simulink model "HVDC_VSC_1CPUcore_dcpl"  (Simulink 8.4)
settings: Solver=ode3  SolverMode=SingleTasking  StartTime=0.0  StopTime=70.0  FixedStep=Ts_Power  RelTol=1e-3  AbsTol=1e-2
PreLoadFcn:
  | Ts_Power=50e-6; Ts_Control=1*Ts_Power; init_cosim_IA; startup_transients_hvdc_vsc;
PostLoadFcn:
  | Ts_Power=50e-6; Ts_Control=1*Ts_Power; init_cosim_IA; startup_transients_hvdc_vsc;
InitFcn:
  | Ts_Power=50e-6; Ts_Control=1*Ts_Power; init_cosim_IA; startup_transients_hvdc_vsc;
values from neighbouring files (symbols this model uses):
  h = 5    [init_cosim_IA.m]
  intfDelay = 400.0    (= 400)    [init_cosim_IA.m]
  Ts_intf = 2*Ts_Power    [init_cosim_IA.m]
undefined symbols (not defined in the file or in its folder): CLARK, D1, Delta, dPref1_2, dPref1_2_rlimit, gcbh, level, lib_mesures, magnitude, ResistanceM, rte_drive_private_lib, rte_tsb3level_hiz_rect_cb, sps_rtmsupport, t_deblock_Pref1, t_deblock_Udref2, t_dPref1_2, t_init_AC, t_SwitchITMIdc, t_SwitchITMVdc, t_vsag_end, t_vsag_start, TSB3_hiZR
libraries: powerlib x162, powerlib_extras x71, spsVIMeasurementModel x63, rteventslib x26, op_dpl_lib x14, powerlib_meascontrol x14, rtlab x6, sps_avr x3, artemis x1
(part 2 of 11)

== system HVDC_VSC_1CPUcore_dcpl/SM_HVDC_VSC/37.5-km  cable ==
  Artemis DPL1 : Subsystem
  Artemis DPL2 : Subsystem
  BI : Subsystem  Tag=ARTEMIS model
      settings: AttributesFormatString=%<Tag>
  PM1 : PMIOPort  Port=1  Side=Left
  PM2 : PMIOPort  Port=2  Side=Right
  wires:
  Artemis DPL2/1(ho) -> Artemis DPL1/1(hi)
  Artemis DPL1/1(ho) -> Artemis DPL2/1(hi)
  connections:
  Artemis DPL2/LConn1 -- PM2/RConn1
  PM1/RConn1 -- Artemis DPL1/LConn1

== system HVDC_VSC_1CPUcore_dcpl/SM_HVDC_VSC/37.5-km  cable1 ==
  Artemis DPL1 : Subsystem
  Artemis DPL2 : Subsystem
  BI : Subsystem  Tag=ARTEMIS model
      settings: AttributesFormatString=%<Tag>
  PM1 : PMIOPort  Port=1  Side=Left
  PM2 : PMIOPort  Port=2  Side=Right
  wires:
  Artemis DPL1/1(ho) -> Artemis DPL2/1(hi)
  Artemis DPL2/1(ho) -> Artemis DPL1/1(hi)
  connections:
  PM1/RConn1 -- Artemis DPL1/LConn1
  Artemis DPL2/LConn1 -- PM2/RConn1

== system HVDC_VSC_1CPUcore_dcpl/SM_HVDC_VSC/37.5-km cable ==
  Artemis DPL1 : Subsystem
  Artemis DPL2 : Subsystem
  BI : Subsystem  Tag=ARTEMIS model
      settings: AttributesFormatString=%<Tag>
  PM1 : PMIOPort  Port=1  Side=Left
  PM2 : PMIOPort  Port=2  Side=Right
  wires:
  Artemis DPL1/1(ho) -> Artemis DPL2/1(hi)
  Artemis DPL2/1(ho) -> Artemis DPL1/1(hi)
  connections:
  PM1/RConn1 -- Artemis DPL1/LConn1
  Artemis DPL2/LConn1 -- PM2/RConn1

== system HVDC_VSC_1CPUcore_dcpl/SM_HVDC_VSC/37.5-km cable1 ==
  Artemis DPL1 : Subsystem
  Artemis DPL2 : Subsystem
  BI : Subsystem  Tag=ARTEMIS model
      settings: AttributesFormatString=%<Tag>
  PM1 : PMIOPort  Port=1  Side=Left
  PM2 : PMIOPort  Port=2  Side=Right
  wires:
  Artemis DPL2/1(ho) -> Artemis DPL1/1(hi)
  Artemis DPL1/1(ho) -> Artemis DPL2/1(hi)
  connections:
  Artemis DPL2/LConn1 -- PM2/RConn1
  PM1/RConn1 -- Artemis DPL1/LConn1

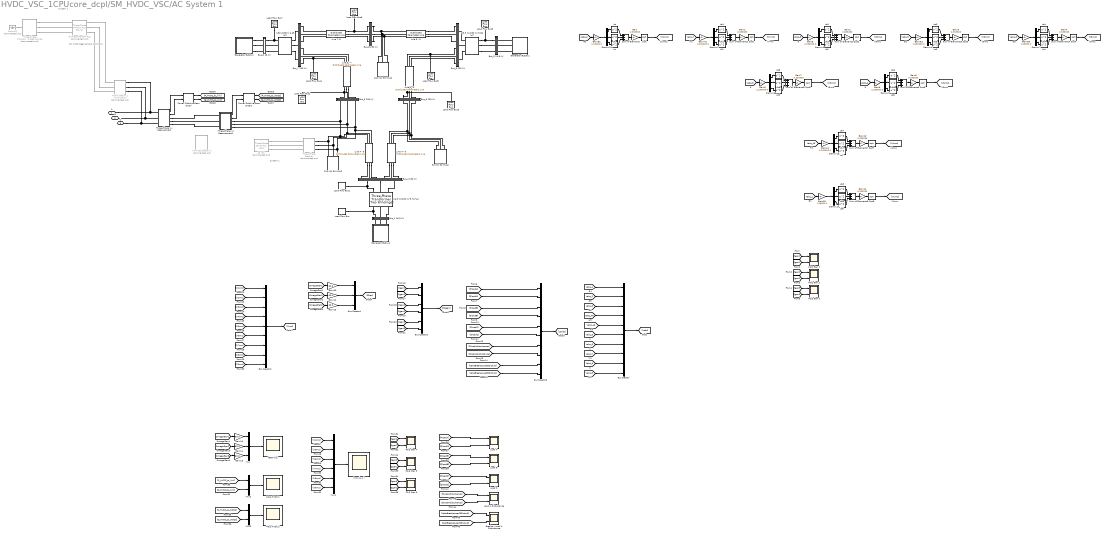
== system HVDC_VSC_1CPUcore_dcpl/SM_HVDC_VSC/AC System 1 ==
  note: phi = 80 (deg) at 1st & 3rd harm.
  note: System 1
  note: System 1
  " Line 4 - 6" : op_dpl_lib/Distributed Parameters Line  SimulationMode=ARTEMIS model  Phases=3  Frequency=60  Resistance=[0.08993 0.224825]  Inductance="[1.41e-3  3.22e-3]"  Capacitance=[7.922e-9 4.74e-9]  Length=100  Measurements=None
  " Line 6 - 9" : op_dpl_lib/Distributed Parameters Line  SimulationMode=ARTEMIS model  Phases=3  Frequency=60  Resistance=[0.20631 0.5157]  Inductance="[2.38e-3  6.09e-3]"  Capacitance=[17.95e-9 10.55e-9]  Length=100  Measurements=None
  100 MW 35 MVAR : powerlib/Elements/Three-Phase Series RLC Load  LConnTagsString=A|B|C  Configuration=Y (grounded)  NominalVoltage=(230000)*1.01601  NominalFrequency=60  ActivePower=100e6  InductivePower=35e6  CapacitivePower=0  Measurements=None  LoadType=constant PQ
  125 MW 50 MVAR : powerlib/Elements/Three-Phase Series RLC Load  LConnTagsString=A|B|C  Configuration=Y (grounded)  NominalVoltage=(230000)*0.996126  NominalFrequency=60  ActivePower=125e6  InductivePower=50e6  CapacitivePower=0  Measurements=None  LoadType=constant PQ
  13.8 KV/230 KV 5.86 %Z : powerlib/Elements/Three-Phase Transformer (Two Windings)  Winding1Connection=Yg  UNITS=pu  NominalPower=[ 128e6 , 60 ]  Winding1=[ 13.8e3 , 1e-6 , 0.0 ]  Winding2Connection=Yg  Winding2=[ 230e3 , 1e-6, 0.075008 ]  SetSaturation=off  Rm=inf  Lm=inf  Saturation=[ 0,0 ; 0.0024,1.2 ; 1.0,1.52 ]  Hysteresis=off  DataFile='hysteresis'  SetInitialFlux=off  InitialFluxes=[ 0.8 , -0.8 , 0.7 ]  Measurements=None  MoreParameters=off  BreakLoop=off  DataType=off  TransfoNumber=1
  "16.5 KV/230 KV 5.76 %Z     " : powerlib/Elements/Three-Phase Transformer (Two Windings)  Winding1Connection=Yg  UNITS=pu  NominalPower=[ 247.5e6 , 60 ]  Winding1=[ 16.5e3 , 1e-6, 0.0 ]  Winding2Connection=Yg  Winding2=[ 230e3 ,1e-6, 0.14256 ]  SetSaturation=off  Rm=inf  Lm=inf  Saturation=[ 0,0 ; 0.0024,1.2 ; 1.0,1.52 ]  Hysteresis=off  DataFile='hysteresis'  SetInitialFlux=off  InitialFluxes=[ 0.8 , -0.8 , 0.7 ]  Measurements=None  MoreParameters=off  BreakLoop=off  DataType=off  TransfoNumber=1
  18KV/230KV 6.25 %Z : powerlib/Elements/Three-Phase Transformer (Two Windings)  Winding1Connection=Yg  UNITS=pu  NominalPower=[ 192e6 , 60 ]  Winding1=[ 18e3 , 1e-6 , 0.0 ]  Winding2Connection=Yg  Winding2=[ 230e3 , 1e-6, 0.12 ]  SetSaturation=off  Rm=inf  Lm=inf  Saturation=[ 0,0 ; 0.0024,1.2 ; 1.0,1.52 ]  Hysteresis=off  DataFile='hysteresis'  SetInitialFlux=off  InitialFluxes=[ 0.8 , -0.8 , 0.7 ]  Measurements=None  MoreParameters=off  BreakLoop=off  DataType=off  TransfoNumber=1
  25 MW : powerlib/Elements/Three-Phase Series RLC Load  Commented=on  LConnTagsString=A|B|C  Configuration=Y (grounded)  NominalVoltage=230000  NominalFrequency=60  ActivePower=25e6  InductivePower=0  CapacitivePower=0  Measurements=None  LoadType=constant PQ
  3- Phase Parallel RLC : powerlib/Elements/Three-Phase Parallel RLC Branch  Commented=on  LConnTagsString=A|B|C  RConnTagsString=A|B|C  BranchType=RL  Resistance=13.79  Inductance=31.02e-3  Capacitance=1.0  Measurements=None
  90 MW 30 MVAR : powerlib/Elements/Three-Phase Series RLC Load  LConnTagsString=A|B|C  Configuration=Y (grounded)  NominalVoltage=(230000)*1.01311  NominalFrequency=60  ActivePower=90e6  InductivePower=30e6  CapacitivePower=0  Measurements=None  LoadType=constant PQ
  Breaker - Load A Disturbance : Scope  NumInputPorts=2
      settings: YMin=110~-1e-13  YMax=110.6~1e-13  SaveName=ScopeData23  Decimation=10
  Bus Creator : BusCreator  Inputs=10
  Bus Creator1 : BusCreator  Inputs=9
  Bus Creator2 : BusCreator  Inputs=6
  Bus Creator3 : BusCreator  Inputs=10
  Bus Creator4 : BusCreator  Inputs=3
  Bus_1 16.5 KV : Subsystem  DialogController=POWERSYS.PowerSysDialog  LoadFcn=sps_rtmsupport('LoadFcn',gcbh);  StartFcn=sps_rtmsupport('StartFcn',gcbh);  StopFcn=sps_rtmsupport('StopFcn',gcbh);  mask(Three-Phase VI Measurement){VoltageMeasurement=phase-to-phase, SetLabelV=on, LabelV=Vabc_1, Vpu=off, VpuLL=off, CurrentMeasurement=yes, SetLabelI=on, LabelI=Iabc_1, Ipu=off, Pbase=100e6, Vbase=16.5e3, OutputType=Complex, PhasorSimulation=off, PSBequivalent=0}
      mask prompts: VoltageMeasurement "Voltage measurement"; SetLabelV "Use a label"; LabelV "Signal label  (use a From block to collect this signal)"; Vpu "Voltages in pu,  based on peak value of nominal phase-to-ground voltage"; VpuLL "Voltages in pu,  based on peak value of nominal phase-to-phase  voltage"; CurrentMeasurement "Current measurement"; SetLabelI "Use a label"; LabelI "Signal label  (use a From block to collect this signal)"; Ipu "Currents in pu"; Pbase "Base power ( VA 3 phase)"; Vbase "Nominal voltage used for pu measurement (Vrms phase-phase) :"; OutputType "Output signals in:"; PhasorSimulation "Phasor simulation (internal use)"; PSBequivalent "Equivalent circuit (internal use)"
      mask help:
      | Ideal three-phase voltage and current measurements.
      |
      | The block can output the voltages and currents in per unit values or in volts and amperes.
      mask init: same as HVDC_VSC_1CPUcore_dcpl/SM_HVDC_VSC/B1
      settings: CopyFcn=sps_rtmsupport('CopyFcn',gcbh); powericon('ThreePhaseVIMeasurementCopy',gcb)  DeleteFcn=sps_rtmsupport('DeleteFcn',gcbh);  UndoDeleteFcn=sps_rtmsupport('UndoDeleteFcn',gcbh);  ModelCloseFcn=sps_rtmsupport('ModelCloseFcn',gcbh);  PreSaveFcn="sps_rtmsupport('PreSaveFcn',gcbh);  set_param(gcb,'LinkStatus','restore')"  PostSaveFcn=sps_rtmsupport('PostSaveFcn',gcbh);  NameChangeFcn=sps_rtmsupport('NameChangeFcn',gcbh);  PreCopyFcn=sps_rtmsupport('PreCopyFcn',gcbh);  OpenFcn=sps_rtmsupport('OpenFcn',gcbh, [1 2 4 5 6 7 9 -12 13]);  CloseFcn=sps_rtmsupport('CloseFcn',gcbh);  PreDeleteFcn=sps_rtmsupport('PreDeleteFcn',gcbh);
      mask Help: helpview(psbhelp)
      mask TypeOptions VoltageMeasurement: no | phase-to-ground | phase-to-phase
      mask Callback VoltageMeasurement: powericon('ThreePhaseVIMeasurementCback',gcb,'Vselector');
      mask Callback SetLabelV: powericon('ThreePhaseVIMeasurementCback',gcb,'');
      mask Callback Vpu: powericon('ThreePhaseVIMeasurementCback',gcb,'Vpu');
      mask Callback VpuLL: powericon('ThreePhaseVIMeasurementCback',gcb,'VpuLL');
      mask TypeOptions CurrentMeasurement: no | yes
      mask Callback CurrentMeasurement: powericon('ThreePhaseVIMeasurementCback',gcb,'');
      mask Callback SetLabelI: powericon('ThreePhaseVIMeasurementCback',gcb,'');
      mask Callback LabelI: powericon('ThreePhaseVIMeasurementCback',gcb,'');
      mask Callback Ipu: powericon('ThreePhaseVIMeasurementCback',gcb,'');
      mask TypeOptions OutputType: Complex | Real-Imag | Magnitude-Angle | Magnitude
  Bus_2 18 KV : Subsystem  DialogController=POWERSYS.PowerSysDialog  LoadFcn=sps_rtmsupport('LoadFcn',gcbh);  StartFcn=sps_rtmsupport('StartFcn',gcbh);  StopFcn=sps_rtmsupport('StopFcn',gcbh);  mask(Three-Phase VI Measurement){VoltageMeasurement=phase-to-phase, SetLabelV=on, LabelV=Vabc_2, Vpu=off, VpuLL=off, CurrentMeasurement=yes, SetLabelI=on, LabelI=Iabc_2, Ipu=off, Pbase=100e6, Vbase=18e3, OutputType=Complex, PhasorSimulation=off, PSBequivalent=0}
      mask prompts: VoltageMeasurement "Voltage measurement"; SetLabelV "Use a label"; LabelV "Signal label  (use a From block to collect this signal)"; Vpu "Voltages in pu,  based on peak value of nominal phase-to-ground voltage"; VpuLL "Voltages in pu,  based on peak value of nominal phase-to-phase  voltage"; CurrentMeasurement "Current measurement"; SetLabelI "Use a label"; LabelI "Signal label  (use a From block to collect this signal)"; Ipu "Currents in pu"; Pbase "Base power ( VA 3 phase)"; Vbase "Nominal voltage used for pu measurement (Vrms phase-phase) :"; OutputType "Output signals in:"; PhasorSimulation "Phasor simulation (internal use)"; PSBequivalent "Equivalent circuit (internal use)"
      mask help:
      | Ideal three-phase voltage and current measurements.
      |
      | The block can output the voltages and currents in per unit values or in volts and amperes.
      mask init: same as HVDC_VSC_1CPUcore_dcpl/SM_HVDC_VSC/B1
      settings: CopyFcn=sps_rtmsupport('CopyFcn',gcbh); powericon('ThreePhaseVIMeasurementCopy',gcb)  DeleteFcn=sps_rtmsupport('DeleteFcn',gcbh);  UndoDeleteFcn=sps_rtmsupport('UndoDeleteFcn',gcbh);  ModelCloseFcn=sps_rtmsupport('ModelCloseFcn',gcbh);  PreSaveFcn="sps_rtmsupport('PreSaveFcn',gcbh);  set_param(gcb,'LinkStatus','restore')"  PostSaveFcn=sps_rtmsupport('PostSaveFcn',gcbh);  NameChangeFcn=sps_rtmsupport('NameChangeFcn',gcbh);  PreCopyFcn=sps_rtmsupport('PreCopyFcn',gcbh);  OpenFcn=sps_rtmsupport('OpenFcn',gcbh, [1 2 4 5 6 7 9 -12 13]);  CloseFcn=sps_rtmsupport('CloseFcn',gcbh);  PreDeleteFcn=sps_rtmsupport('PreDeleteFcn',gcbh);
      mask Help: helpview(psbhelp)
      mask TypeOptions VoltageMeasurement: no | phase-to-ground | phase-to-phase
      mask Callback VoltageMeasurement: powericon('ThreePhaseVIMeasurementCback',gcb,'Vselector');
      mask Callback SetLabelV: powericon('ThreePhaseVIMeasurementCback',gcb,'');
      mask Callback Vpu: powericon('ThreePhaseVIMeasurementCback',gcb,'Vpu');
      mask Callback VpuLL: powericon('ThreePhaseVIMeasurementCback',gcb,'VpuLL');
      mask TypeOptions CurrentMeasurement: no | yes
      mask Callback CurrentMeasurement: powericon('ThreePhaseVIMeasurementCback',gcb,'');
      mask Callback SetLabelI: powericon('ThreePhaseVIMeasurementCback',gcb,'');
      mask Callback LabelI: powericon('ThreePhaseVIMeasurementCback',gcb,'');
      mask Callback Ipu: powericon('ThreePhaseVIMeasurementCback',gcb,'');
      mask TypeOptions OutputType: Complex | Real-Imag | Magnitude-Angle | Magnitude
  Bus_3 13.8 KV : Subsystem  DialogController=POWERSYS.PowerSysDialog  LoadFcn=sps_rtmsupport('LoadFcn',gcbh);  StartFcn=sps_rtmsupport('StartFcn',gcbh);  StopFcn=sps_rtmsupport('StopFcn',gcbh);  mask(Three-Phase VI Measurement){VoltageMeasurement=phase-to-phase, SetLabelV=on, LabelV=Vabc_3, Vpu=off, VpuLL=off, CurrentMeasurement=yes, SetLabelI=on, LabelI=Iabc_3, Ipu=off, Pbase=100e6, Vbase=13.8e3, OutputType=Complex, PhasorSimulation=off, PSBequivalent=0}
      mask prompts: VoltageMeasurement "Voltage measurement"; SetLabelV "Use a label"; LabelV "Signal label  (use a From block to collect this signal)"; Vpu "Voltages in pu,  based on peak value of nominal phase-to-ground voltage"; VpuLL "Voltages in pu,  based on peak value of nominal phase-to-phase  voltage"; CurrentMeasurement "Current measurement"; SetLabelI "Use a label"; LabelI "Signal label  (use a From block to collect this signal)"; Ipu "Currents in pu"; Pbase "Base power ( VA 3 phase)"; Vbase "Nominal voltage used for pu measurement (Vrms phase-phase) :"; OutputType "Output signals in:"; PhasorSimulation "Phasor simulation (internal use)"; PSBequivalent "Equivalent circuit (internal use)"
      mask help:
      | Ideal three-phase voltage and current measurements.
      |
      | The block can output the voltages and currents in per unit values or in volts and amperes.
      mask init: same as HVDC_VSC_1CPUcore_dcpl/SM_HVDC_VSC/B1
      settings: CopyFcn=sps_rtmsupport('CopyFcn',gcbh); powericon('ThreePhaseVIMeasurementCopy',gcb)  DeleteFcn=sps_rtmsupport('DeleteFcn',gcbh);  UndoDeleteFcn=sps_rtmsupport('UndoDeleteFcn',gcbh);  ModelCloseFcn=sps_rtmsupport('ModelCloseFcn',gcbh);  PreSaveFcn="sps_rtmsupport('PreSaveFcn',gcbh);  set_param(gcb,'LinkStatus','restore')"  PostSaveFcn=sps_rtmsupport('PostSaveFcn',gcbh);  NameChangeFcn=sps_rtmsupport('NameChangeFcn',gcbh);  PreCopyFcn=sps_rtmsupport('PreCopyFcn',gcbh);  OpenFcn=sps_rtmsupport('OpenFcn',gcbh, [1 2 4 5 6 7 9 -12 13]);  CloseFcn=sps_rtmsupport('CloseFcn',gcbh);  PreDeleteFcn=sps_rtmsupport('PreDeleteFcn',gcbh);
      mask Help: helpview(psbhelp)
      mask TypeOptions VoltageMeasurement: no | phase-to-ground | phase-to-phase
      mask Callback VoltageMeasurement: powericon('ThreePhaseVIMeasurementCback',gcb,'Vselector');
      mask Callback SetLabelV: powericon('ThreePhaseVIMeasurementCback',gcb,'');
      mask Callback Vpu: powericon('ThreePhaseVIMeasurementCback',gcb,'Vpu');
      mask Callback VpuLL: powericon('ThreePhaseVIMeasurementCback',gcb,'VpuLL');
      mask TypeOptions CurrentMeasurement: no | yes
      mask Callback CurrentMeasurement: powericon('ThreePhaseVIMeasurementCback',gcb,'');
      mask Callback SetLabelI: powericon('ThreePhaseVIMeasurementCback',gcb,'');
      mask Callback LabelI: powericon('ThreePhaseVIMeasurementCback',gcb,'');
      mask Callback Ipu: powericon('ThreePhaseVIMeasurementCback',gcb,'');
      mask TypeOptions OutputType: Complex | Real-Imag | Magnitude-Angle | Magnitude
  Bus_4 230 KV : Subsystem
  Bus_5 230 KV : Subsystem  DialogController=POWERSYS.PowerSysDialog  LoadFcn=sps_rtmsupport('LoadFcn',gcbh);  StartFcn=sps_rtmsupport('StartFcn',gcbh);  StopFcn=sps_rtmsupport('StopFcn',gcbh);  mask(Three-Phase VI Measurement){VoltageMeasurement=phase-to-phase, SetLabelV=on, LabelV=Vabc_5, Vpu=off, VpuLL=off, CurrentMeasurement=yes, SetLabelI=on, LabelI=Iabc_5, Ipu=off, Pbase=100e6, Vbase=230e3, OutputType=Complex, PhasorSimulation=off, PSBequivalent=0}
      mask prompts: VoltageMeasurement "Voltage measurement"; SetLabelV "Use a label"; LabelV "Signal label  (use a From block to collect this signal)"; Vpu "Voltages in pu,  based on peak value of nominal phase-to-ground voltage"; VpuLL "Voltages in pu,  based on peak value of nominal phase-to-phase  voltage"; CurrentMeasurement "Current measurement"; SetLabelI "Use a label"; LabelI "Signal label  (use a From block to collect this signal)"; Ipu "Currents in pu"; Pbase "Base power ( VA 3 phase)"; Vbase "Nominal voltage used for pu measurement (Vrms phase-phase) :"; OutputType "Output signals in:"; PhasorSimulation "Phasor simulation (internal use)"; PSBequivalent "Equivalent circuit (internal use)"
      mask help:
      | Ideal three-phase voltage and current measurements.
      |
      | The block can output the voltages and currents in per unit values or in volts and amperes.
      mask init: same as HVDC_VSC_1CPUcore_dcpl/SM_HVDC_VSC/B1
      settings: CopyFcn=sps_rtmsupport('CopyFcn',gcbh); powericon('ThreePhaseVIMeasurementCopy',gcb)  DeleteFcn=sps_rtmsupport('DeleteFcn',gcbh);  UndoDeleteFcn=sps_rtmsupport('UndoDeleteFcn',gcbh);  ModelCloseFcn=sps_rtmsupport('ModelCloseFcn',gcbh);  PreSaveFcn="sps_rtmsupport('PreSaveFcn',gcbh);  set_param(gcb,'LinkStatus','restore')"  PostSaveFcn=sps_rtmsupport('PostSaveFcn',gcbh);  NameChangeFcn=sps_rtmsupport('NameChangeFcn',gcbh);  PreCopyFcn=sps_rtmsupport('PreCopyFcn',gcbh);  OpenFcn=sps_rtmsupport('OpenFcn',gcbh, [1 2 4 5 6 7 9 -12 13]);  CloseFcn=sps_rtmsupport('CloseFcn',gcbh);  PreDeleteFcn=sps_rtmsupport('PreDeleteFcn',gcbh);
      mask Help: helpview(psbhelp)
      mask TypeOptions VoltageMeasurement: no | phase-to-ground | phase-to-phase
      mask Callback VoltageMeasurement: powericon('ThreePhaseVIMeasurementCback',gcb,'Vselector');
      mask Callback SetLabelV: powericon('ThreePhaseVIMeasurementCback',gcb,'');
      mask Callback Vpu: powericon('ThreePhaseVIMeasurementCback',gcb,'Vpu');
      mask Callback VpuLL: powericon('ThreePhaseVIMeasurementCback',gcb,'VpuLL');
      mask TypeOptions CurrentMeasurement: no | yes
      mask Callback CurrentMeasurement: powericon('ThreePhaseVIMeasurementCback',gcb,'');
      mask Callback SetLabelI: powericon('ThreePhaseVIMeasurementCback',gcb,'');
      mask Callback LabelI: powericon('ThreePhaseVIMeasurementCback',gcb,'');
      mask Callback Ipu: powericon('ThreePhaseVIMeasurementCback',gcb,'');
      mask TypeOptions OutputType: Complex | Real-Imag | Magnitude-Angle | Magnitude
  Bus_6 230 KV : Subsystem  DialogController=POWERSYS.PowerSysDialog  LoadFcn=sps_rtmsupport('LoadFcn',gcbh);  StartFcn=sps_rtmsupport('StartFcn',gcbh);  StopFcn=sps_rtmsupport('StopFcn',gcbh);  mask(Three-Phase VI Measurement){VoltageMeasurement=phase-to-phase, SetLabelV=on, LabelV=Vabc_6, Vpu=off, VpuLL=off, CurrentMeasurement=yes, SetLabelI=on, LabelI=Iabc_6, Ipu=off, Pbase=100e6, Vbase=230e3, OutputType=Complex, PhasorSimulation=off, PSBequivalent=0}
      mask prompts: VoltageMeasurement "Voltage measurement"; SetLabelV "Use a label"; LabelV "Signal label  (use a From block to collect this signal)"; Vpu "Voltages in pu,  based on peak value of nominal phase-to-ground voltage"; VpuLL "Voltages in pu,  based on peak value of nominal phase-to-phase  voltage"; CurrentMeasurement "Current measurement"; SetLabelI "Use a label"; LabelI "Signal label  (use a From block to collect this signal)"; Ipu "Currents in pu"; Pbase "Base power ( VA 3 phase)"; Vbase "Nominal voltage used for pu measurement (Vrms phase-phase) :"; OutputType "Output signals in:"; PhasorSimulation "Phasor simulation (internal use)"; PSBequivalent "Equivalent circuit (internal use)"
      mask help:
      | Ideal three-phase voltage and current measurements.
      |
      | The block can output the voltages and currents in per unit values or in volts and amperes.
      mask init: same as HVDC_VSC_1CPUcore_dcpl/SM_HVDC_VSC/B1
      settings: CopyFcn=sps_rtmsupport('CopyFcn',gcbh); powericon('ThreePhaseVIMeasurementCopy',gcb)  DeleteFcn=sps_rtmsupport('DeleteFcn',gcbh);  UndoDeleteFcn=sps_rtmsupport('UndoDeleteFcn',gcbh);  ModelCloseFcn=sps_rtmsupport('ModelCloseFcn',gcbh);  PreSaveFcn="sps_rtmsupport('PreSaveFcn',gcbh);  set_param(gcb,'LinkStatus','restore')"  PostSaveFcn=sps_rtmsupport('PostSaveFcn',gcbh);  NameChangeFcn=sps_rtmsupport('NameChangeFcn',gcbh);  PreCopyFcn=sps_rtmsupport('PreCopyFcn',gcbh);  OpenFcn=sps_rtmsupport('OpenFcn',gcbh, [1 2 4 5 6 7 9 -12 13]);  CloseFcn=sps_rtmsupport('CloseFcn',gcbh);  PreDeleteFcn=sps_rtmsupport('PreDeleteFcn',gcbh);
      mask Help: helpview(psbhelp)
      mask TypeOptions VoltageMeasurement: no | phase-to-ground | phase-to-phase
      mask Callback VoltageMeasurement: powericon('ThreePhaseVIMeasurementCback',gcb,'Vselector');
      mask Callback SetLabelV: powericon('ThreePhaseVIMeasurementCback',gcb,'');
      mask Callback Vpu: powericon('ThreePhaseVIMeasurementCback',gcb,'Vpu');
      mask Callback VpuLL: powericon('ThreePhaseVIMeasurementCback',gcb,'VpuLL');
      mask TypeOptions CurrentMeasurement: no | yes
      mask Callback CurrentMeasurement: powericon('ThreePhaseVIMeasurementCback',gcb,'');
      mask Callback SetLabelI: powericon('ThreePhaseVIMeasurementCback',gcb,'');
      mask Callback LabelI: powericon('ThreePhaseVIMeasurementCback',gcb,'');
      mask Callback Ipu: powericon('ThreePhaseVIMeasurementCback',gcb,'');
      mask TypeOptions OutputType: Complex | Real-Imag | Magnitude-Angle | Magnitude
  Bus_7 230 KV : Subsystem
  Bus_8 230 KV : Subsystem  DialogController=POWERSYS.PowerSysDialog  LoadFcn=sps_rtmsupport('LoadFcn',gcbh);  StartFcn=sps_rtmsupport('StartFcn',gcbh);  StopFcn=sps_rtmsupport('StopFcn',gcbh);  mask(Three-Phase VI Measurement){VoltageMeasurement=phase-to-phase, SetLabelV=on, LabelV=Vabc_8, Vpu=off, VpuLL=off, CurrentMeasurement=yes, SetLabelI=on, LabelI=Iabc_8, Ipu=off, Pbase=100e6, Vbase=230e3, OutputType=Complex, PhasorSimulation=off, PSBequivalent=0}
      mask prompts: VoltageMeasurement "Voltage measurement"; SetLabelV "Use a label"; LabelV "Signal label  (use a From block to collect this signal)"; Vpu "Voltages in pu,  based on peak value of nominal phase-to-ground voltage"; VpuLL "Voltages in pu,  based on peak value of nominal phase-to-phase  voltage"; CurrentMeasurement "Current measurement"; SetLabelI "Use a label"; LabelI "Signal label  (use a From block to collect this signal)"; Ipu "Currents in pu"; Pbase "Base power ( VA 3 phase)"; Vbase "Nominal voltage used for pu measurement (Vrms phase-phase) :"; OutputType "Output signals in:"; PhasorSimulation "Phasor simulation (internal use)"; PSBequivalent "Equivalent circuit (internal use)"
      mask help:
      | Ideal three-phase voltage and current measurements.
      |
      | The block can output the voltages and currents in per unit values or in volts and amperes.
      mask init: same as HVDC_VSC_1CPUcore_dcpl/SM_HVDC_VSC/B1
      settings: CopyFcn=sps_rtmsupport('CopyFcn',gcbh); powericon('ThreePhaseVIMeasurementCopy',gcb)  DeleteFcn=sps_rtmsupport('DeleteFcn',gcbh);  UndoDeleteFcn=sps_rtmsupport('UndoDeleteFcn',gcbh);  ModelCloseFcn=sps_rtmsupport('ModelCloseFcn',gcbh);  PreSaveFcn="sps_rtmsupport('PreSaveFcn',gcbh);  set_param(gcb,'LinkStatus','restore')"  PostSaveFcn=sps_rtmsupport('PostSaveFcn',gcbh);  NameChangeFcn=sps_rtmsupport('NameChangeFcn',gcbh);  PreCopyFcn=sps_rtmsupport('PreCopyFcn',gcbh);  OpenFcn=sps_rtmsupport('OpenFcn',gcbh, [1 2 4 5 6 7 9 -12 13]);  CloseFcn=sps_rtmsupport('CloseFcn',gcbh);  PreDeleteFcn=sps_rtmsupport('PreDeleteFcn',gcbh);
      mask Help: helpview(psbhelp)
      mask TypeOptions VoltageMeasurement: no | phase-to-ground | phase-to-phase
      mask Callback VoltageMeasurement: powericon('ThreePhaseVIMeasurementCback',gcb,'Vselector');
      mask Callback SetLabelV: powericon('ThreePhaseVIMeasurementCback',gcb,'');
      mask Callback Vpu: powericon('ThreePhaseVIMeasurementCback',gcb,'Vpu');
      mask Callback VpuLL: powericon('ThreePhaseVIMeasurementCback',gcb,'VpuLL');
      mask TypeOptions CurrentMeasurement: no | yes
      mask Callback CurrentMeasurement: powericon('ThreePhaseVIMeasurementCback',gcb,'');
      mask Callback SetLabelI: powericon('ThreePhaseVIMeasurementCback',gcb,'');
      mask Callback LabelI: powericon('ThreePhaseVIMeasurementCback',gcb,'');
      mask Callback Ipu: powericon('ThreePhaseVIMeasurementCback',gcb,'');
      mask TypeOptions OutputType: Complex | Real-Imag | Magnitude-Angle | Magnitude
  Bus_9 230 KV : Subsystem
  Demux{2..4,6..7,9..10,17,24} (9 alike) : Demux  Outputs=3
  Gain{,1..4,7,9..11} (9 alike) : Gain  Gain=0.333333
  Gain{12..16,60} (6 alike) : Gain  Gain=60.0
  Gain4/1 : Gain  Gain=1/230000.0
  Gain5 : Gain  Gain=1/230000.0
  Gain6 : Gain  Gain=1/230000.0
  Gain7/1 : Gain  Gain=1/230000.0
  Gain8 : Gain  Gain=1/230000.0
  Gain9/1 : Gain  Gain=1/230000.0
  GainG1 : Gain  Gain=1/16500.0
  GainG2 : Gain  Gain=1/18000.0
  GainG3 : Gain  Gain=1/13800.0
  Generator BUS1x1 : Subsystem
  Generator BUS2x1 : Subsystem
  Generator BUS3x1 : Subsystem
  Ground2 : powerlib/Elements/Ground  Commented=on  LConnTagsString=a
  HVDC Station 1 Initialization : powerlib/Elements/Three-Phase Breaker  Commented=on  InitialState=closed  SwitchA=on  SwitchB=on  SwitchC=on  SwitchTimes=[ 11.5 ]  External=off  BreakerResistance=0.01  SnubberResistance=1e6  SnubberCapacitance=inf  Measurements=None
  "Line 4 - 5 " : op_dpl_lib/Distributed Parameters Line  SimulationMode=ARTEMIS model  Phases=3  Frequency=60  Resistance=[0.0529 0.13225]  Inductance="[1.2599e-3  2.38e-3]"  Capacitance=[8.82e-9 5.188e-9]  Length=100  Measurements=None
  "Line 5 - 7 " : op_dpl_lib/Distributed Parameters Line  SimulationMode=ARTEMIS model  Phases=3  Frequency=60  Resistance=[0.16928 0.4232]  Inductance="[2.259e-3  5.64e-3]"  Capacitance=[15.34e-9 9.025e-9]  Length=100  Measurements=None
  Line 7- 8 : op_dpl_lib/Distributed Parameters Line  SimulationMode=ARTEMIS model  Phases=3  Frequency=60  Resistance=[0.044965 0.8768175]  Inductance=[1.488e-3 1.488e-3]  Capacitance=[7.471e-9 7.471e-9]  Length=100  Measurements=None
  Line 8 - 9 : op_dpl_lib/Distributed Parameters Line  SimulationMode=ARTEMIS model  Phases=3  Frequency=60  Resistance=[0.062951 0.15737]  Inductance="[1.414e-3  3.53e-3]"  Capacitance=[10.47e-9 6.15e-9]  Length=100  Measurements=None
  Load A : Scope  NumInputPorts=2
      settings: YMin=1.06e+08~4.6e+07  YMax=1.26e+08~5.05e+07  SaveName=ScopeData33  Decimation=10
  Load A Disturbance : Scope  NumInputPorts=2
      settings: YMin=110~-1e-13  YMax=110.6~1e-13  SaveName=ScopeData34  Decimation=10
  Load B : Scope  NumInputPorts=2
      settings: YMin=8.95e+07~2.96e+07  YMax=9.04e+07~3.02e+07  SaveName=ScopeData35  Decimation=10
  Load C : Scope  NumInputPorts=2
      settings: YMin=9.95e+07~3.46e+07  YMax=1.005e+08~3.53e+07  SaveName=ScopeData36  Decimation=10
  Load Flow Bus : powerlib/Measurements/Load Flow Bus  LConnTagsString=a  ID=BUS_1  Vbase=16.5e3  Vref=1.04  Vangle=0  VLF=1.04  angleLF=0
      settings: AttributesFormatString=%<ID>\n%<Vbase>V\n%<VLF>pu\n%<angleLF>deg.
  Load Flow Bus1 : powerlib/Measurements/Load Flow Bus  LConnTagsString=a  ID=BUS_4  Vbase=230e3  Vref=1  Vangle=0  VLF=1.026  angleLF=-2.214
      settings: AttributesFormatString=%<ID>\n%<Vbase>V\n%<VLF>pu\n%<angleLF>deg.
  Load Flow Bus2 : powerlib/Measurements/Load Flow Bus  LConnTagsString=a  ID=BUS_5  Vbase=230e3  Vref=1  Vangle=0  VLF=0.9961  angleLF=-3.98
      settings: AttributesFormatString=%<ID>\n%<Vbase>V\n%<VLF>pu\n%<angleLF>deg.
  Load Flow Bus3 : powerlib/Measurements/Load Flow Bus  LConnTagsString=a  ID=BUS_6  Vbase=230e3  Vref=1  Vangle=0  VLF=1.013  angleLF=-3.678
      settings: AttributesFormatString=%<ID>\n%<Vbase>V\n%<VLF>pu\n%<angleLF>deg.
  Load Flow Bus4 : powerlib/Measurements/Load Flow Bus  LConnTagsString=a  ID=BUS_7  Vbase=230e3  Vref=1  Vangle=0  VLF=1.026  angleLF=3.662
      settings: AttributesFormatString=%<ID>\n%<Vbase>V\n%<VLF>pu\n%<angleLF>deg.
  Load Flow Bus5 : powerlib/Measurements/Load Flow Bus  LConnTagsString=a  ID=BUS_9  Vbase=230e3  Vref=1  Vangle=0  VLF=1.032  angleLF=1.909
      settings: AttributesFormatString=%<ID>\n%<Vbase>V\n%<VLF>pu\n%<angleLF>deg.
  Load Flow Bus6 : powerlib/Measurements/Load Flow Bus  LConnTagsString=a  ID=BUS_8  Vbase=230e3  Vref=1  Vangle=0  VLF=1.016  angleLF=0.6755
      settings: AttributesFormatString=%<ID>\n%<Vbase>V\n%<VLF>pu\n%<angleLF>deg.
  Load Flow Bus7 : powerlib/Measurements/Load Flow Bus  LConnTagsString=a  ID=BUS_2  Vbase=18e3  Vref=1.025  Vangle=0  VLF=1.025  angleLF=9.222
      settings: AttributesFormatString=%<ID>\n%<Vbase>V\n%<VLF>pu\n%<angleLF>deg.
  Load Flow Bus8 : powerlib/Measurements/Load Flow Bus  LConnTagsString=a  ID=BUS_3  Vbase=13.8e3  Vref=1.025  Vangle=4.7  VLF=1.025  angleLF=4.606
      settings: AttributesFormatString=%<ID>\n%<Vbase>V\n%<VLF>pu\n%<angleLF>deg.
  Mux : Mux  Inputs=3
  Mux1 : Mux  Inputs=6
  Mux2 : Mux  Inputs=2
  Mux3 : Mux  Inputs=2
  P&Q Gen {1..6} (6 alike) : Scope  NumInputPorts=2
      P&Q Gen 1 settings: YMin=6e+07~-1.5e+08  YMax=2.2e+08~2e+08  SaveName=ScopeData7  Decimation=10
      P&Q Gen 2 settings: YMin=1.626e+08~5.9e+06  YMax=1.642e+08~6.7e+06  SaveName=ScopeData8  Decimation=10
      P&Q Gen 3 settings: YMin=8.46e+07~-1.115e+07  YMax=8.58e+07~-1.065e+07  SaveName=ScopeData9  Decimation=10
      P&Q Gen 4 settings: YMin=6e+07~-1.5e+08  YMax=2.4e+08~2e+08  SaveName=ScopeData10  Decimation=10
      P&Q Gen 5 settings: YMin=1.2e+08~-8e+07  YMax=3.2e+08~2e+07  SaveName=ScopeData15  Decimation=10
      P&Q Gen 6 settings: YMin=8.46e+07~-1.115e+07  YMax=8.58e+07~-1.065e+07  SaveName=ScopeData22  Decimation=10
  P&Q HVDC 1 : Scope
      settings: ShowLegends=on  YMin=-2.5e+08  YMax=2.5e+08  SaveName=ScopeData11
  P&Q HVDC 2 : Scope
      settings: ShowLegends=on  YMin=-2.5e+08  YMax=2.5e+08  SaveName=ScopeData12
  Power (Positive-Sequence) : powerlib_meascontrol/Measurements/Power (Positive-Sequence)  Freq=60  Vinit=[0, 0]  Iinit=[0, 0]  Ts=0
  Power (Positive-Sequence)1 : powerlib_meascontrol/Measurements/Power (Positive-Sequence)  Freq=60  Vinit=[0, 0]  Iinit=[0, 0]  Ts=0
  Sqrt{,1..8} (9 alike) : Sqrt  SaturateOnIntegerOverflow=on
  Sum of Elements{,1..8} (9 alike) : Sum  Inputs=+|+|+
  Three-Phase Programmable Voltage Source : powerlib/Electrical Sources/Three-Phase Programmable Voltage Source  Commented=on  PositiveSequence="[230e3  0  60]"  VariationEntity=None  VariationType=Step  VariationTypeAlt=Step  VariationStep=vsag_mag  VariationRate=10  VariationMagnitude=0.3  VariationFrequency=2  VariationTiming="[t_vsag_start  t_vsag_end]"  VariationPhaseA=off  Amplitudes=[1 0.8 1.2 1.0]  TimeValues=[0 0.1 0.15 0.2]  HarmonicGeneration=off  HarmonicA="[2 0.10  0  2]"  HarmonicB="[2  0  35 2]"  Timing="[1.2  99]"  BusType=swing  Pref=0  Qref=0  Qmin=-inf  Qmax=inf
  Three-Phase V-I Measurement : Subsystem  DialogController=POWERSYS.PowerSysDialog  LoadFcn=sps_rtmsupport('LoadFcn',gcbh);  StartFcn=sps_rtmsupport('StartFcn',gcbh);  StopFcn=sps_rtmsupport('StopFcn',gcbh);  mask(Three-Phase VI Measurement){VoltageMeasurement=phase-to-ground, SetLabelV=off, LabelV=Vabc, Vpu=off, VpuLL=off, CurrentMeasurement=yes, SetLabelI=off, LabelI=Iabc, Ipu=off, Pbase=100e6, Vbase=500e3, OutputType=Complex, PhasorSimulation=off, PSBequivalent=0}
      mask prompts: VoltageMeasurement "Voltage measurement"; SetLabelV "Use a label"; LabelV "Signal label  (use a From block to collect this signal)"; Vpu "Voltages in pu,  based on peak value of nominal phase-to-ground voltage"; VpuLL "Voltages in pu,  based on peak value of nominal phase-to-phase  voltage"; CurrentMeasurement "Current measurement"; SetLabelI "Use a label"; LabelI "Signal label  (use a From block to collect this signal)"; Ipu "Currents in pu"; Pbase "Base power ( VA 3 phase)"; Vbase "Nominal voltage used for pu measurement (Vrms phase-phase) :"; OutputType "Output signals in:"; PhasorSimulation "Phasor simulation (internal use)"; PSBequivalent "Equivalent circuit (internal use)"
      mask help:
      | Ideal three-phase voltage and current measurements.
      |
      | The block can output the voltages and currents in per unit values or in volts and amperes.
      mask init: same as HVDC_VSC_1CPUcore_dcpl/SM_HVDC_VSC/B1
      settings: CopyFcn=sps_rtmsupport('CopyFcn',gcbh); powericon('ThreePhaseVIMeasurementCopy',gcb)  DeleteFcn=sps_rtmsupport('DeleteFcn',gcbh);  UndoDeleteFcn=sps_rtmsupport('UndoDeleteFcn',gcbh);  ModelCloseFcn=sps_rtmsupport('ModelCloseFcn',gcbh);  PreSaveFcn="sps_rtmsupport('PreSaveFcn',gcbh);  set_param(gcb,'LinkStatus','restore')"  PostSaveFcn=sps_rtmsupport('PostSaveFcn',gcbh);  NameChangeFcn=sps_rtmsupport('NameChangeFcn',gcbh);  PreCopyFcn=sps_rtmsupport('PreCopyFcn',gcbh);  OpenFcn=sps_rtmsupport('OpenFcn',gcbh, [1 2 4 5 6 7 9 -12 13]);  CloseFcn=sps_rtmsupport('CloseFcn',gcbh);  PreDeleteFcn=sps_rtmsupport('PreDeleteFcn',gcbh);
      mask Help: helpview(psbhelp)
      mask TypeOptions VoltageMeasurement: no | phase-to-ground | phase-to-phase
      mask Callback VoltageMeasurement: powericon('ThreePhaseVIMeasurementCback',gcb,'Vselector');
      mask Callback SetLabelV: powericon('ThreePhaseVIMeasurementCback',gcb,'');
      mask Callback Vpu: powericon('ThreePhaseVIMeasurementCback',gcb,'Vpu');
      mask Callback VpuLL: powericon('ThreePhaseVIMeasurementCback',gcb,'VpuLL');
      mask TypeOptions CurrentMeasurement: no | yes
      mask Callback CurrentMeasurement: powericon('ThreePhaseVIMeasurementCback',gcb,'');
      mask Callback SetLabelI: powericon('ThreePhaseVIMeasurementCback',gcb,'');
      mask Callback LabelI: powericon('ThreePhaseVIMeasurementCback',gcb,'');
      mask Callback Ipu: powericon('ThreePhaseVIMeasurementCback',gcb,'');
      mask TypeOptions OutputType: Complex | Real-Imag | Magnitude-Angle | Magnitude
  Three-Phase V-I Measurement1 : Subsystem  DialogController=POWERSYS.PowerSysDialog  LoadFcn=sps_rtmsupport('LoadFcn',gcbh);  StartFcn=sps_rtmsupport('StartFcn',gcbh);  StopFcn=sps_rtmsupport('StopFcn',gcbh);  mask(Three-Phase VI Measurement){VoltageMeasurement=phase-to-ground, SetLabelV=off, LabelV=Vabc, Vpu=off, VpuLL=off, CurrentMeasurement=yes, SetLabelI=off, LabelI=Iabc, Ipu=off, Pbase=100e6, Vbase=500e3, OutputType=Complex, PhasorSimulation=off, PSBequivalent=0}
      mask prompts: VoltageMeasurement "Voltage measurement"; SetLabelV "Use a label"; LabelV "Signal label  (use a From block to collect this signal)"; Vpu "Voltages in pu,  based on peak value of nominal phase-to-ground voltage"; VpuLL "Voltages in pu,  based on peak value of nominal phase-to-phase  voltage"; CurrentMeasurement "Current measurement"; SetLabelI "Use a label"; LabelI "Signal label  (use a From block to collect this signal)"; Ipu "Currents in pu"; Pbase "Base power ( VA 3 phase)"; Vbase "Nominal voltage used for pu measurement (Vrms phase-phase) :"; OutputType "Output signals in:"; PhasorSimulation "Phasor simulation (internal use)"; PSBequivalent "Equivalent circuit (internal use)"
      mask help:
      | Ideal three-phase voltage and current measurements.
      |
      | The block can output the voltages and currents in per unit values or in volts and amperes.
      mask init: same as HVDC_VSC_1CPUcore_dcpl/SM_HVDC_VSC/B1
      settings: CopyFcn=sps_rtmsupport('CopyFcn',gcbh); powericon('ThreePhaseVIMeasurementCopy',gcb)  DeleteFcn=sps_rtmsupport('DeleteFcn',gcbh);  UndoDeleteFcn=sps_rtmsupport('UndoDeleteFcn',gcbh);  ModelCloseFcn=sps_rtmsupport('ModelCloseFcn',gcbh);  PreSaveFcn="sps_rtmsupport('PreSaveFcn',gcbh);  set_param(gcb,'LinkStatus','restore')"  PostSaveFcn=sps_rtmsupport('PostSaveFcn',gcbh);  NameChangeFcn=sps_rtmsupport('NameChangeFcn',gcbh);  PreCopyFcn=sps_rtmsupport('PreCopyFcn',gcbh);  OpenFcn=sps_rtmsupport('OpenFcn',gcbh, [1 2 4 5 6 7 9 -12 13]);  CloseFcn=sps_rtmsupport('CloseFcn',gcbh);  PreDeleteFcn=sps_rtmsupport('PreDeleteFcn',gcbh);
      mask Help: helpview(psbhelp)
      mask TypeOptions VoltageMeasurement: no | phase-to-ground | phase-to-phase
      mask Callback VoltageMeasurement: powericon('ThreePhaseVIMeasurementCback',gcb,'Vselector');
      mask Callback SetLabelV: powericon('ThreePhaseVIMeasurementCback',gcb,'');
      mask Callback Vpu: powericon('ThreePhaseVIMeasurementCback',gcb,'Vpu');
      mask Callback VpuLL: powericon('ThreePhaseVIMeasurementCback',gcb,'VpuLL');
      mask TypeOptions CurrentMeasurement: no | yes
      mask Callback CurrentMeasurement: powericon('ThreePhaseVIMeasurementCback',gcb,'');
      mask Callback SetLabelI: powericon('ThreePhaseVIMeasurementCback',gcb,'');
      mask Callback LabelI: powericon('ThreePhaseVIMeasurementCback',gcb,'');
      mask Callback Ipu: powericon('ThreePhaseVIMeasurementCback',gcb,'');
      mask TypeOptions OutputType: Complex | Real-Imag | Magnitude-Angle | Magnitude
  Three-Phase Breaker : powerlib/Elements/Three-Phase Breaker  Commented=on  InitialState=open  SwitchA=on  SwitchB=on  SwitchC=on  SwitchTimes=[ 50.0 ]  External=off  BreakerResistance=0.01  SnubberResistance=1e6  SnubberCapacitance=inf  Measurements=Breaker voltages and currents
  To HVDC Station 1 : powerlib/Elements/Three-Phase Breaker  Commented=on  InitialState=open  SwitchA=on  SwitchB=on  SwitchC=on  SwitchTimes=[ t_init_AC ]  External=off  BreakerResistance=0.01  SnubberResistance=1e6  SnubberCapacitance=inf  Measurements=None
  Ua{,1..8} (9 alike) : Math  Operator=square  SaturateOnIntegerOverflow=on
  Ub{,1..8} (9 alike) : Math  Operator=square  SaturateOnIntegerOverflow=on
  Uc{,1..8} (9 alike) : Math  Operator=square  SaturateOnIntegerOverflow=on
  Vrms (p.u.) : Scope
      settings: ShowLegends=on  YMin=0.6  YMax=1.8  SaveName=ScopeData17
  fGEN [Hz] : Scope
      settings: YMin=59.2  YMax=60.4  SaveName=ScopeData16
  A : PMIOPort  Port=1  Side=Right
  B : PMIOPort  Port=2  Side=Right
  C : PMIOPort  Port=3  Side=Right
  wires:
  Bus Creator2/1 -> [PQgen]
  Bus Creator/1 -> [Vabc]
  [Vabc_5] -> Gain5/1
  [Vabc_7] -> Gain7/1/1
  [Vabc_45] -> Gain4/1/1
  GainG2/1 -> Demux24/1
  [Vabc_2] -> GainG2/1
  [Vabc_6] -> Gain6/1
  [Vabc_8] -> Gain8/1
  [Vabc_3] -> GainG3/1
  [Vabc_1] -> GainG1/1
  [Vabc_9] -> Gain9/1/1
  Demux3/1 -> Ua2/1
  Ub/1 -> Sum of Elements/2
  Uc1/1 -> Sum of Elements1/3
  Ua4/1 -> Sum of Elements4/1
  Gain5/1 -> Demux6/1
  Demux2/2 -> Ub1/1
  Gain4/1 -> Sqrt4/1
  Gain7/1/1 -> Demux2/1
  Ub1/1 -> Sum of Elements1/2
  Demux6/1 -> Ua5/1
  Demux2/3 -> Uc1/1
  Sqrt/1 -> [V2rms]
  Gain/1 -> Sqrt/1
  Sqrt1/1 -> [V7rms]
  Demux3/3 -> Uc2/1
  Demux24/2 -> Ub/1
  Uc/1 -> Sum of Elements/3
  Ua/1 -> Sum of Elements/1
  Ub3/1 -> Sum of Elements3/2
  Gain1/1 -> Sqrt1/1
  Demux24/3 -> Uc/1
  Demux2/1 -> Ua1/1
  Ua1/1 -> Sum of Elements1/1
  Sum of Elements/1 -> Gain/1
  Gain8/1 -> Demux3/1
  Demux7/3 -> Uc4/1
  Gain3/1 -> Sqrt3/1
  Sum of Elements1/1 -> Gain1/1
  Demux24/1 -> Ua/1
  Gain6/1 -> Demux9/1
  Demux6/3 -> Uc5/1
  Uc4/1 -> Sum of Elements4/3
  Demux6/2 -> Ub5/1
  Demux4/2 -> Ub3/1
  Demux7/1 -> Ua4/1
  Demux7/2 -> Ub4/1
  Sqrt2/1 -> [V8rms]
  Demux4/1 -> Ua3/1
  Gain2/1 -> Sqrt2/1
  Uc3/1 -> Sum of Elements3/3
  Ua3/1 -> Sum of Elements3/1
  Demux3/2 -> Ub2/1
  GainG3/1 -> Demux7/1
  Uc2/1 -> Sum of Elements2/3
  Gain9/1/1 -> Demux4/1
  Sum of Elements3/1 -> Gain3/1
  Ua5/1 -> Sum of Elements5/1
  Ub4/1 -> Sum of Elements4/2
  Sum of Elements4/1 -> Gain4/1
  Sqrt3/1 -> [V9rms]
  Ub2/1 -> Sum of Elements2/2
  Sum of Elements2/1 -> Gain2/1
  Demux4/3 -> Uc3/1
  Demux9/2 -> Ub6/1
  Sqrt7/1 -> [V4rms]
  Ub5/1 -> Sum of Elements5/2
  Ua2/1 -> Sum of Elements2/1
  Ua6/1 -> Sum of Elements6/1
  Sum of Elements6/1 -> Gain9/1
  GainG1/1 -> Demux17/1
  Gain10/1 -> Sqrt7/1
  Sum of Elements7/1 -> Gain10/1
  Gain9/1 -> Sqrt6/1
  Ua7/1 -> Sum of Elements7/1
  Demux10/1 -> Ua7/1
  Demux17/3 -> Uc8/1
  Ub6/1 -> Sum of Elements6/2
  Demux9/1 -> Ua6/1
  Ub8/1 -> Sum of Elements8/2
  Demux10/2 -> Ub7/1
  Sum of Elements8/1 -> Gain11/1
  Uc6/1 -> Sum of Elements6/3
  Demux9/3 -> Uc6/1
  Demux10/3 -> Uc7/1
  Ub7/1 -> Sum of Elements7/2
  Uc8/1 -> Sum of Elements8/3
  Uc7/1 -> Sum of Elements7/3
  Uc5/1 -> Sum of Elements5/3
  Sqrt6/1 -> [V6rms]
  Demux17/1 -> Ua8/1
  Demux17/2 -> Ub8/1
  Sum of Elements5/1 -> Gain7/1
  Ua8/1 -> Sum of Elements8/1
  Gain11/1 -> Sqrt8/1
  Gain7/1 -> Sqrt5/1
  Sqrt8/1 -> [V1rms]
  Gain4/1/1 -> Demux10/1
  Sqrt4/1 -> [V3rms]
  Sqrt5/1 -> [V5rms]
  Bus Creator3/1 -> [Loads]
  [V1rms] -> Bus Creator1/1  "V1rms"
  [V3rms] -> Bus Creator1/3  "V3rms"
  [V4rms] -> Bus Creator1/4  "V4rms"
  [V2rms] -> Bus Creator1/2  "V2rms"
  [V7rms] -> Bus Creator1/7  "V7rms"
  [V5rms] -> Bus Creator1/5  "V5rms"
  [V6rms] -> Bus Creator1/6  "V6rms"
  [Vabc_9] -> Bus Creator/10  "Vabc_9"
  [Vabc_7] -> Bus Creator/8  "Vabc_7"
  [Vabc_8] -> Bus Creator/9  "Vabc_8"
  [Vabc_3] -> Bus Creator/3  "Vabc_3"
  [Vabc_5] -> Bus Creator/6  "Vabc_5"
  [Vabc_6] -> Bus Creator/7  "Vabc_6"
  [Vabc_46] -> Bus Creator/5  "Vabc_46"
  [Vabc_2] -> Bus Creator/2  "Vabc_2"
  [Vabc_45] -> Bus Creator/4  "Vabc_45"
  [Vabc_1] -> Bus Creator/1  "Vabc_1"
  [Qgen2] -> P&Q Gen 2/2
  [Pgen3] -> P&Q Gen 3/1
  [Pgen2] -> P&Q Gen 2/1
  [Qgen3] -> P&Q Gen 3/2
  [Qgen1] -> P&Q Gen 1/2
  [Pgen1] -> P&Q Gen 1/1
  [PloadAdisturbance] -> Bus Creator3/7  "PloadAdisturbance"
  [PloadB] -> Bus Creator3/3  "PloadB"
  [QloadB] -> Bus Creator3/4  "QloadB"
  [QloadAdisturbance] -> Bus Creator3/8  "QloadAdisturbance"
  [QloadC] -> Bus Creator3/6  "QloadC"
  [PloadC] -> Bus Creator3/5  "PloadC"
  [QloadA] -> Bus Creator3/2  "QloadA"
  [IabcBreakerLoad5Disturb] -> Bus Creator3/10  "IabcBreakerLoad5Disturb"
  [UabcBreakerLoad5Disturb] -> Bus Creator3/9  "UabcBreakerLoad5Disturb"
  [PloadA] -> Bus Creator3/1  "PloadA"
  [Qgen3] -> Bus Creator2/6  "Qgen3"
  [Pgen2] -> Bus Creator2/3  "Pgen2"
  [Pgen3] -> Bus Creator2/5  "Pgen3"
  [Qgen1] -> Bus Creator2/2  "Qgen1"
  [Pgen1] -> Bus Creator2/1  "Pgen1"
  [Qgen2] -> Bus Creator2/4  "Qgen2"
  Bus Creator1/1 -> [Vrms]
  [V9rms] -> Bus Creator1/9  "V9rms"
  [V8rms] -> Bus Creator1/8  "V8rms"
  Bus Creator4/1 -> [fGen]
  [OmegaGen1] -> Gain60/1
  [OmegaGen2] -> Gain12/1
  [OmegaGen3] -> Gain13/1
  Gain60/1 -> Bus Creator4/1  "fGen1"
  Gain12/1 -> Bus Creator4/2  "fGen2"
  Gain13/1 -> Bus Creator4/3  "fGen3"
  [V4rms] -> Mux1/1
  Mux/1 -> fGEN [Hz]/1
  [V7rms] -> Mux1/4
  [V9rms] -> Mux1/6
  [V6rms] -> Mux1/3
  [V5rms] -> Mux1/2
  [V8rms] -> Mux1/5
  Mux1/1 -> Vrms (p.u.)/1
  [Pgen3] -> P&Q Gen 6/1
  [Qgen1] -> P&Q Gen 4/2
  [Qgen2] -> P&Q Gen 5/2
  [Pgen1] -> P&Q Gen 4/1
  [Pgen2] -> P&Q Gen 5/1
  [Qgen3] -> P&Q Gen 6/2
  [PloadA] -> Load A/1
  [QloadA] -> Load A/2
  [PloadB] -> Load B/1
  [QloadB] -> Load B/2
  [PloadC] -> Load C/1
  [QloadC] -> Load C/2
  [PloadAdisturbance] -> Load A Disturbance/1
  [QloadAdisturbance] -> Load A Disturbance/2
  [IabcBreakerLoad5Disturb] -> Breaker - Load A Disturbance/2
  [UabcBreakerLoad5Disturb] -> Breaker - Load A Disturbance/1
  [OmegaGen1] -> Gain16/1
  [OmegaGen2] -> Gain14/1
  [OmegaGen3] -> Gain15/1
  Gain16/1 -> Mux/1
  Gain14/1 -> Mux/2
  Gain15/1 -> Mux/3
  Three-Phase V-I Measurement/2(Iabc) -> Power (Positive-Sequence)/2
  Three-Phase V-I Measurement/1(Vabc) -> Power (Positive-Sequence)/1
  Power (Positive-Sequence)/1 -> [P_HVDC_to_link]
  [P_HVDC_to_link] -> Mux2/1
  [Q_HVDC_to_link] -> Mux2/2
  Mux2/1 -> P&Q HVDC 1/1
  [P_HVDC_to_WSCC] -> Mux3/1
  [Q_HVDC_to_WSCC] -> Mux3/2
  Mux3/1 -> P&Q HVDC 2/1
  Three-Phase V-I Measurement1/2(Iabc) -> Power (Positive-Sequence)1/2
  Three-Phase V-I Measurement1/1(Vabc) -> Power (Positive-Sequence)1/1
  Power (Positive-Sequence)/2 -> [Q_HVDC_to_link]
  Power (Positive-Sequence)1/1 -> [P_HVDC_to_WSCC]
  Power (Positive-Sequence)1/2 -> [Q_HVDC_to_WSCC]
  connections:
  Three-Phase Programmable Voltage Source/RConn1 -- 3- Phase Parallel RLC/LConn1
  Three-Phase Programmable Voltage Source/RConn2 -- 3- Phase Parallel RLC/LConn2
  Three-Phase Programmable Voltage Source/RConn3 -- 3- Phase Parallel RLC/LConn3
  Ground2/LConn1 -- Three-Phase Programmable Voltage Source/LConn1
  Bus_3 13.8 KV/LConn1 -- Load Flow Bus8/LConn1 -- 13.8 KV/230 KV 5.86 %Z/LConn1
  "16.5 KV/230 KV 5.76 %Z     "/RConn1 -- Bus_4 230 KV/LConn1 -- Load Flow Bus1/LConn1
  "16.5 KV/230 KV 5.76 %Z     "/LConn1 -- Bus_1 16.5 KV/LConn1 -- Load Flow Bus/LConn1
  18KV/230KV 6.25 %Z/LConn1 -- Bus_2 18 KV/RConn1 -- Load Flow Bus7/LConn1
  Bus_8 230 KV/LConn3 -- 100 MW 35 MVAR/LConn3 -- Line 8 - 9/LConn3
  Load Flow Bus3/LConn1 -- Bus_6 230 KV/LConn1 -- " Line 6 - 9"/RConn1
  Load Flow Bus6/LConn1 -- Bus_8 230 KV/RConn1 -- Line 7- 8/RConn1
  125 MW 50 MVAR/LConn3 -- Three-Phase Breaker/RConn3 -- "Line 4 - 5 "/LConn3 -- Three-Phase V-I Measurement1/RConn3 -- Bus_5 230 KV/RConn3
  Bus_7 230 KV/RConn6 -- Load Flow Bus4/LConn1 -- "Line 5 - 7 "/LConn1
  125 MW 50 MVAR/LConn2 -- Three-Phase Breaker/RConn2 -- "Line 4 - 5 "/LConn2 -- Three-Phase V-I Measurement1/RConn2 -- Bus_5 230 KV/RConn2
  " Line 6 - 9"/LConn1 -- Load Flow Bus5/LConn1 -- Bus_9 230 KV/LConn4
  125 MW 50 MVAR/LConn1 -- Three-Phase Breaker/RConn1 -- "Line 4 - 5 "/LConn1 -- Three-Phase V-I Measurement1/RConn1 -- Bus_5 230 KV/RConn1
  Bus_8 230 KV/LConn2 -- 100 MW 35 MVAR/LConn2 -- Line 8 - 9/LConn2
  Bus_6 230 KV/RConn2 -- 90 MW 30 MVAR/LConn2 -- " Line 4 - 6"/LConn2
  Bus_8 230 KV/LConn1 -- 100 MW 35 MVAR/LConn1 -- Line 8 - 9/LConn1
  Bus_6 230 KV/RConn1 -- 90 MW 30 MVAR/LConn1 -- " Line 4 - 6"/LConn1
  Bus_6 230 KV/RConn3 -- 90 MW 30 MVAR/LConn3 -- " Line 4 - 6"/LConn3
  Load Flow Bus2/LConn1 -- "Line 5 - 7 "/RConn1 -- Bus_5 230 KV/LConn1
  13.8 KV/230 KV 5.86 %Z/LConn2 -- Bus_3 13.8 KV/LConn2
  Bus_1 16.5 KV/LConn2 -- "16.5 KV/230 KV 5.76 %Z     "/LConn2
  13.8 KV/230 KV 5.86 %Z/RConn3 -- Bus_9 230 KV/RConn3
  Generator BUS1x1/RConn3 -- Bus_1 16.5 KV/RConn3
  Bus_1 16.5 KV/LConn3 -- "16.5 KV/230 KV 5.76 %Z     "/LConn3
  Bus_4 230 KV/LConn2 -- "16.5 KV/230 KV 5.76 %Z     "/RConn2
  13.8 KV/230 KV 5.86 %Z/LConn3 -- Bus_3 13.8 KV/LConn3
  Line 7- 8/RConn2 -- Bus_8 230 KV/RConn2
  Line 7- 8/RConn3 -- Bus_8 230 KV/RConn3
  " Line 6 - 9"/RConn2 -- Bus_6 230 KV/LConn2
  " Line 6 - 9"/LConn2 -- Bus_9 230 KV/LConn5
  Generator BUS1x1/RConn1 -- Bus_1 16.5 KV/RConn1
  18KV/230KV 6.25 %Z/LConn2 -- Bus_2 18 KV/RConn2
  "Line 5 - 7 "/RConn3 -- Bus_5 230 KV/LConn3
  13.8 KV/230 KV 5.86 %Z/RConn1 -- Bus_9 230 KV/RConn1
  13.8 KV/230 KV 5.86 %Z/RConn2 -- Bus_9 230 KV/RConn2
  Generator BUS2x1/RConn2 -- Bus_2 18 KV/LConn2
  Generator BUS1x1/RConn2 -- Bus_1 16.5 KV/RConn2
  Bus_2 18 KV/RConn3 -- 18KV/230KV 6.25 %Z/LConn3
  "Line 5 - 7 "/LConn3 -- Bus_7 230 KV/RConn4
  Generator BUS3x1/RConn3 -- Bus_3 13.8 KV/RConn3
  18KV/230KV 6.25 %Z/RConn1 -- Bus_7 230 KV/LConn1
  Line 7- 8/LConn3 -- Bus_7 230 KV/RConn3
  " Line 4 - 6"/RConn2 -- Bus_4 230 KV/RConn5
  "Line 4 - 5 "/RConn3 -- Bus_4 230 KV/RConn3
  "Line 4 - 5 "/RConn2 -- Bus_4 230 KV/RConn2
  "Line 5 - 7 "/RConn2 -- Bus_5 230 KV/LConn2
  25 MW/LConn2 -- Three-Phase Breaker/LConn2
  Line 8 - 9/RConn3 -- Bus_9 230 KV/LConn3
  Line 7- 8/LConn1 -- Bus_7 230 KV/RConn1
  "Line 4 - 5 "/RConn1 -- Bus_4 230 KV/RConn1
  " Line 4 - 6"/RConn3 -- Bus_4 230 KV/RConn6
  "16.5 KV/230 KV 5.76 %Z     "/RConn3 -- Bus_4 230 KV/LConn3
  Generator BUS2x1/RConn3 -- Bus_2 18 KV/LConn3
  25 MW/LConn1 -- Three-Phase Breaker/LConn1
  " Line 6 - 9"/LConn3 -- Bus_9 230 KV/LConn6
  18KV/230KV 6.25 %Z/RConn2 -- Bus_7 230 KV/LConn2
  25 MW/LConn3 -- Three-Phase Breaker/LConn3
  " Line 4 - 6"/RConn1 -- Bus_4 230 KV/RConn4
  Generator BUS2x1/RConn1 -- Bus_2 18 KV/LConn1
  18KV/230KV 6.25 %Z/RConn3 -- Bus_7 230 KV/LConn3
  " Line 6 - 9"/RConn3 -- Bus_6 230 KV/LConn3
  Line 7- 8/LConn2 -- Bus_7 230 KV/RConn2
  Generator BUS3x1/RConn2 -- Bus_3 13.8 KV/RConn2
  Line 8 - 9/RConn2 -- Bus_9 230 KV/LConn2
  Line 8 - 9/RConn1 -- Bus_9 230 KV/LConn1
  "Line 5 - 7 "/LConn2 -- Bus_7 230 KV/RConn5
  Generator BUS3x1/RConn1 -- Bus_3 13.8 KV/RConn1
  3- Phase Parallel RLC/RConn1 -- HVDC Station 1 Initialization/LConn1
  3- Phase Parallel RLC/RConn2 -- HVDC Station 1 Initialization/LConn2
  3- Phase Parallel RLC/RConn3 -- HVDC Station 1 Initialization/LConn3
  A/RConn1 -- HVDC Station 1 Initialization/RConn1 -- Three-Phase V-I Measurement/LConn1
  B/RConn1 -- HVDC Station 1 Initialization/RConn2 -- Three-Phase V-I Measurement/LConn2
  C/RConn1 -- HVDC Station 1 Initialization/RConn3 -- Three-Phase V-I Measurement/LConn3
  Three-Phase V-I Measurement/RConn2 -- Three-Phase V-I Measurement1/LConn2
  Three-Phase V-I Measurement/RConn1 -- Three-Phase V-I Measurement1/LConn1
  Three-Phase V-I Measurement/RConn3 -- Three-Phase V-I Measurement1/LConn3
